simulink model "bh_explore_1dof_on_the_ROAD"  (R2026b)
settings: Solver=ode15s  StopTime=12  MaxStep=0.001  RelTol=1e-5  EnableMultiTasking=on
values from neighbouring files (symbols this model uses):
  s = saveObjectImpl@matlab.System(obj)    [bh_road_hump_A_SYSO.m]
undefined symbols (not defined in the file or in its folder): plant_T, X, Y, Z
libraries: sm_lib x5, nesl_utility x1
settings Model: Creator=smiller  LastModifiedBy=bhorton
settings DataIOCC: LimitDataPoints=on  ReturnWorkspaceOutputs=off  SaveFormat=Array
settings OptimizationCC: LifeSpan=inf
settings DebuggingCC: AllowSymbolicDim=off  ArithmeticOperatorsInVariantConditions=warning  MergeDetectMultiDrivingBlocksExec=none  SFExecutionAtInitializationDiag=none  SFNoUnconditionalDefaultTransitionDiag=warning  SFUnexpectedBacktrackingDiag=warning  SolverPrmCheckMsg=warning  StateNameClashWarn=warning  UnderspecifiedInitializationDetection=Classic
settings HardwareCC: ProdEndianess=Unspecified  ProdHWDeviceType=32-bit Generic  ProdIntDivRoundTo=Undefined  ProdLargestAtomicFloat=None
settings ModelReferenceCC: PropagateSignalLabelsOutOfModel=off
settings SFSimCC: CustomCodeUndefinedFunction=UseInterfaceOnly  SimUseLocalCustomCode=off
settings RTWCC: DLArmComputeVersion=19.05  RTWUseLocalCustomCode=off
settings CodeAppCC: StateflowObjectComments=on
settings GRTTargetCC: TargetLangStandard=C89/C90 (ANSI)
settings ConfigComp: CovExternalEMLEnable=off  CovSFcnEnable=off  CovSaveCumulativeToWorkspaceVar=on  CovSaveSingleToWorkspaceVar=on
settings SimscapeCC: SimscapeNormalizeSystem=off  SimscapeUseEnergyAccounting=off
settings ExplorerConfigSet: InternalSimMechanicsExplorerSettings=|
  | <ExplorerConfiguration>
  | 
  |   <canonicalview>default</canonicalview>
  | 
  |   <TilePanel>
  |     <TileInfo>
  |       <Tiles Columns="1" Count="1" Height="395" Rows="1" Width="675">
  |         <Row Weight="1"/>
  |         <Column Weight="1"/>
  |         <Tile Height="1" Width="1" X="0" Y="0"/>
  |       </Tiles>
  |     </TileInfo>
  |     <SceneInfo>
  |       <SceneViewer>
  |         <IsThisViewStd>
  |           <IsStandardView>off</IsStandardView>
  |           <StandardViewName>Front</StandardViewName>
  |         </IsThisViewStd>
  |         <BGColor>
  |           <R>0.60000002384185791</R>
  |           <G>0.60000002384185791</G>
  |           <B>0.60000002384185791</B>
  |           <A>1</A>
  |         </BGColor>
  |         <Camera>
  |           <DoPerspective>on</DoPerspective>
  |           <Position>
  |             <X>0</X>
  |             <Y>-4.9406564584124654e-324</Y>
  |             <Z>3</Z>
  |           </Position>
  |           <Center>
  |             <X>0</X>
  |             <Y>-4.9406564584124654e-324</Y>
  |             <Z>0</Z>
  |           </Center>
  |           <Up>
  |             <X>0</X>
  |             <Y>1</Y>
  |             <Z>0</Z>
  |           </Up>
  |           <XLim>1.3989229744649958</XLim>
  |           <YLim>1.3989229744649958</YLim>
  |           <ViewLimDist>0.01</ViewLimDist>
  |         </Camera>
  |       </SceneViewer>
  |     </SceneInfo>
  |   </TilePanel>
  | 
  |   <MechEditorPanel>
  |     <GfxPanelCameraMap>
  |       <MapElement CameraMLId="Camera1" GfxPanelIndex="0"/>
  |     </GfxPanelCameraMap>
  |     <Cameras>
  |       <Camera>
  |         <Id>Camera1</Id>
  |         <Value>
  |           <Name>Camera1</Name>
  |           <NativeCamera>
  |             <PositionTrackingFeature>CAR_SIMSCAPE.RF_CAM.R</PositionTrackingFeature>
  |             <CenterTrackingFeature>CAR_SIMSCAPE.Road.R</CenterTrackingFeature>
  |             <UpVectorTrackingFeature>CAR_SIMSCAPE.RF1.R</UpVectorTrackingFeature>
  |             <CenterTrackingOrigin>on</CenterTrackingOrigin>
  |             <UpVectorTrackingDirection>+Y</UpVectorTrackingDirection>
  |           </NativeCamera>
  |         </Value>
  |       </Camera>
  |     </Cameras>
  |     <VideoCreator>
  |       <IncludeTiles>All</IncludeTiles>
  |       <IncludeTime>off</IncludeTime>
  |       <IncludeWorldFrame>off</IncludeWorldFrame>
  |       <PlaybackSpeedRatio>2</PlaybackSpeedRatio>
  |       <FrameRate>30</FrameRate>
  |       <FrameSize>[400, 400]</FrameSize>
  |       <VideoFormat>MPEG4</VideoFormat>
  |     </VideoCreator>
  |   </MechEditorPanel>
  | 
  |   <PlaybackSettings>
  |     <PlaybackSpeedFactor>0.5</PlaybackSpeedFactor>
  |   </PlaybackSettings>
  | 
  | </ExplorerConfiguration>

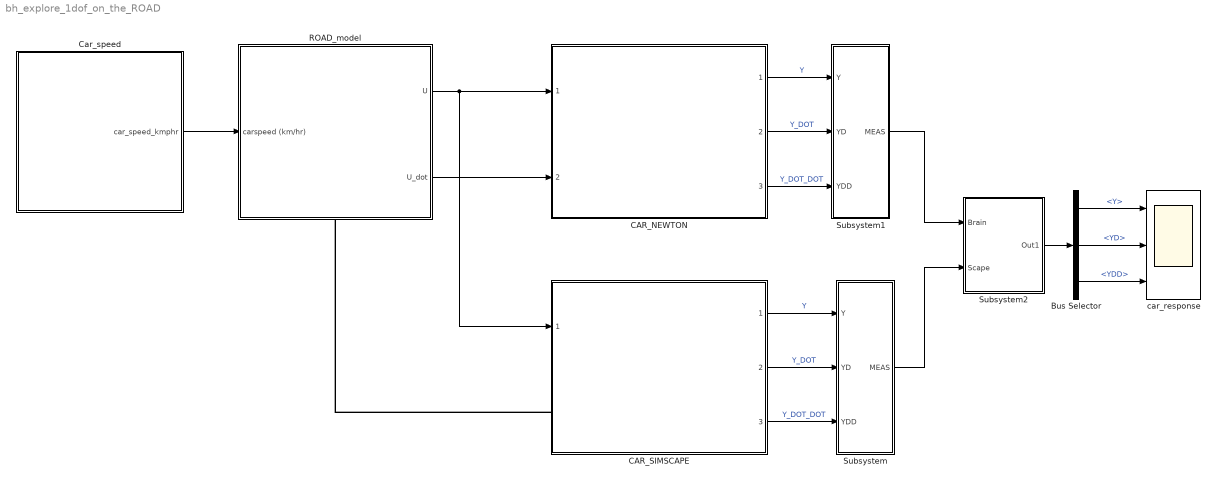
== system bh_explore_1dof_on_the_ROAD ==
  Bus Selector : BusSelector  OutputSignals=Y,YD,YDD
  CAR_NEWTON : Subsystem  ReferencedSubsystem=bh_COMPONENT_1dof_NEWTON  m=plant_T.m  c=plant_T.c  k=plant_T.k  y0=IC_T.y  y_dot_0=IC_T.y_dot
  CAR_SIMSCAPE : Subsystem  ReferencedSubsystem=bh_COMPONENT_1dof_SIMSCAPE  m=plant_T.m  c=plant_T.c  k=plant_T.k  L_EQ=IC_T.L_EQ  U_m_rel_R=IC_T.U_m_rel_R  U_m_rel_R_dot=IC_T.U_m_rel_R_dot
  Car_speed : Subsystem
  ROAD_model : Subsystem
      settings: PortSchema="{\"entries\":[{\"content\":{\"sides\":[{\"content\":{\"connectorIds\":[\"In1\"]},\"type\":\"ConnectorPlacement.EquallySpacedRectSide\",\"uuid\":\"1fb0e359-1d6f-495f-b416-4042b3ceba31\"},{\"content\":{\"connectorIds\":[\"Out1\",\"Out2\"],\"side\":\"RIGHT\"},\"type\":\"ConnectorPlacement.EquallySpacedRectSide\",\"uuid\":\"86004b89-795c-49b7-9809-342f6a5939d0\"},{\"content\":{\"side\":\"TOP\"},\"type\":\"ConnectorPlacement.EquallySpacedRectSide\",\"uuid\":\"63e39511-0cd1-4623-81a4-4c1485d2dba0\"},{\"content\":{\"connectorIds\":[\"RConn1\"],\"side\":\"BOTTOM\"},\"type\":\"ConnectorPlacement.EquallySpacedRectSide\",\"uuid\":\"6d6a2f3b-9911-4ef3-b1fe-c7ef6b98e3da\"}]},\"type\":\"ConnectorPlacement.EquallySpacedConnector\",\"uuid\":\"0b009940-cb7a-402d-bea6-65ae1d55ed5c\"}],\"packageUris\":[\"http://schema.mathworks.com/mf0/Connector/R2020b\"],\"version\":\"1.0\"}"
  Subsystem : Subsystem
  Subsystem1 : Subsystem
  Subsystem2 : Subsystem
  car_response : Scope  NumInputPorts=3
      settings: ActiveDisplayYMinimum=-0.2278214499400405  ActiveDisplayYMaximum=-0.13085171197243853  DataLoggingVariableName=ScopeData2
  wires:
  Car_speed/1(car_speed_kmphr) -> ROAD_model/1(carspeed (km/hr))
  Bus Selector/2 -> car_response/2  "<YD>"
  CAR_SIMSCAPE/2 -> Subsystem/2(YD)  "Y_DOT"
  CAR_NEWTON/1 -> Subsystem1/1(Y)  "Y"
  Subsystem2/1(Out1) -> Bus Selector/1
  Bus Selector/1 -> car_response/1  "<Y>"
  CAR_NEWTON/2 -> Subsystem1/2(YD)  "Y_DOT"
  CAR_SIMSCAPE/3 -> Subsystem/3(YDD)  "Y_DOT_DOT"
  CAR_NEWTON/3 -> Subsystem1/3(YDD)  "Y_DOT_DOT"
  CAR_SIMSCAPE/1 -> Subsystem/1(Y)  "Y"
  Bus Selector/3 -> car_response/3  "<YDD>"
  Subsystem1/1(MEAS) -> Subsystem2/1(Brain)
  Subsystem/1(MEAS) -> Subsystem2/2(Scape)
  ROAD_model/1(U) -> CAR_NEWTON/1, CAR_SIMSCAPE/1
  ROAD_model/2(U_dot) -> CAR_NEWTON/2
  connections:
  CAR_SIMSCAPE/LConn1 -- ROAD_model/RConn1

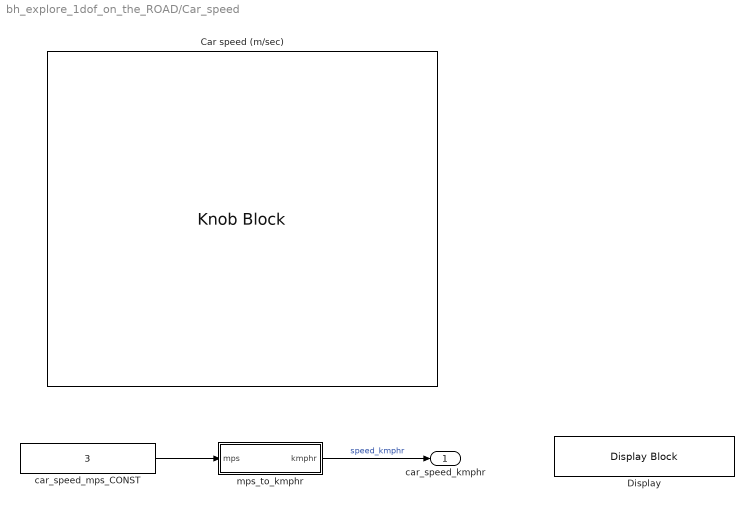
== system bh_explore_1dof_on_the_ROAD/Car_speed ==
  Car speed (m/sec) : KnobBlock  LabelPosition=Hide  ScaleMax=30  TickInterval=1
  Display : DisplayBlock  Transparency=1  GridColor=[0.502, 0.502, 0.502]
  car_speed_mps_CONST : Constant  Value=3
  mps_to_kmphr : Subsystem
  car_speed_kmphr : Outport
  wires:
  car_speed_mps_CONST/1 -> mps_to_kmphr/1(mps)
  mps_to_kmphr/1(kmphr) -> car_speed_kmphr/1  "speed_kmphr"

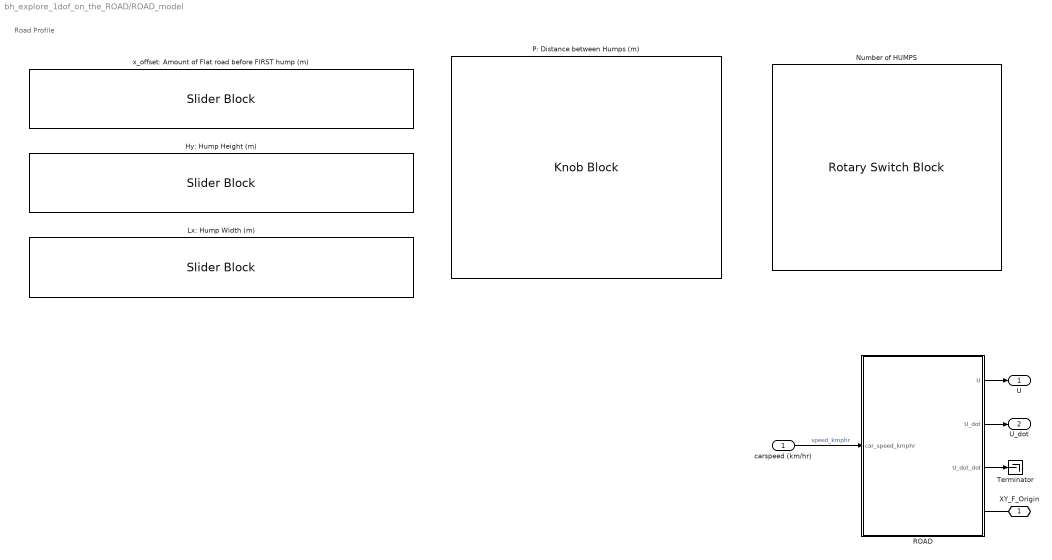
== system bh_explore_1dof_on_the_ROAD/ROAD_model ==
  note: Road Profile
  carspeed (km/hr) : Inport
  Hy: Hump Height (m) : SliderBlock  LabelPosition=Hide  ScaleMax=0.25
  Lx: Hump Width (m) : SliderBlock  LabelPosition=Hide  ScaleMax=1
  Number of HUMPS : RotarySwitchBlock  LabelPosition=Hide
  P: Distance between Humps (m) : KnobBlock  LabelPosition=Hide
  ROAD : Subsystem  mask{m_Hy=0.1981572234156821, m_Lx=1, m_P=9.707276629144626, m_x_offset=2, m_Np=20}
      mask prompts: m_Hy "Height of hump (m)"; m_Lx "Length of hump (m)"; m_P "Period of window (m)"; m_x_offset "X direction offset"; m_Np "Number of periods"
      mask init:
      | % create SYS object
      | OBJ = bh_road_hump_A_SYSO("Hy",m_Hy, "Lx",m_Lx, "P",m_P, ...
      |                           "x_offset",m_x_offset, "NUM_PERIODS",m_Np);
      |                       
      | tmp_x = linspace(0,(m_Np*m_P  +  m_x_offset), 1e4);
      | tmp_y = OBJ.get_y(tmp_x);
      | tmp_z = -2 * ones(size(tmp_x));
      | 
      | the_road_XYZ = [ tmp_x(:), tmp_y(:), tmp_z(:) ];
      mask DialogControl Control2 Prompt: Road Profile Parameters
  Terminator : Terminator
  x_offset: Amount of Flat road before FIRST hump (m) : SliderBlock  LabelPosition=Hide  ScaleMax=10
  XY_F_Origin : PMIOPort  Side=Right
  U : Outport
  U_dot : Outport  Port=2
  wires:
  ROAD/1(U) -> U/1
  ROAD/3(U_dot_dot) -> Terminator/1
  ROAD/2(U_dot) -> U_dot/1
  carspeed (km/hr)/1 -> ROAD/1(car_speed_kmphr)  "speed_kmphr"
  connections:
  XY_F_Origin/RConn1 -- ROAD/RConn1

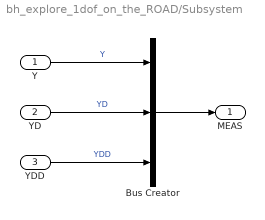
== system bh_explore_1dof_on_the_ROAD/Subsystem ==
  Y : Inport
  YD : Inport  Port=2
  YDD : Inport  Port=3
  Bus Creator : BusCreator  Inputs=3
  MEAS : Outport
  wires:
  YD/1 -> Bus Creator/2  "YD"
  YDD/1 -> Bus Creator/3  "YDD"
  Y/1 -> Bus Creator/1  "Y"
  Bus Creator/1 -> MEAS/1

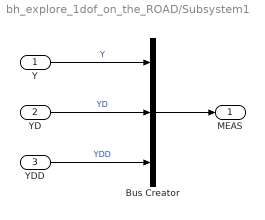
== system bh_explore_1dof_on_the_ROAD/Subsystem1 ==
  Y : Inport
  YD : Inport  Port=2
  YDD : Inport  Port=3
  Bus Creator : BusCreator  Inputs=3
  MEAS : Outport
  wires:
  YD/1 -> Bus Creator/2  "YD"
  YDD/1 -> Bus Creator/3  "YDD"
  Y/1 -> Bus Creator/1  "Y"
  Bus Creator/1 -> MEAS/1

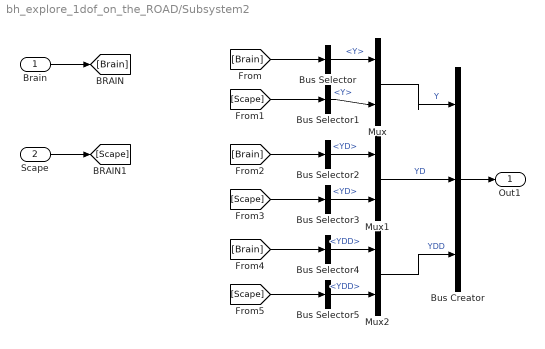
== system bh_explore_1dof_on_the_ROAD/Subsystem2 ==
  Brain : Inport
  Scape : Inport  Port=2
  Bus Creator : BusCreator  Inputs=3
  Bus Selector : BusSelector  OutputSignals=Y
  Bus Selector1 : BusSelector  OutputSignals=Y
  Bus Selector2 : BusSelector  OutputSignals=YD
  Bus Selector3 : BusSelector  OutputSignals=YD
  Bus Selector4 : BusSelector  OutputSignals=YDD
  Bus Selector5 : BusSelector  OutputSignals=YDD
  Mux : Mux  Inputs=2
  Mux1 : Mux  Inputs=2
  Mux2 : Mux  Inputs=2
  Out1 : Outport
  wires:
  Scape/1 -> [Scape]
  Brain/1 -> [Brain]
  [Brain] -> Bus Selector/1
  [Scape] -> Bus Selector1/1
  Bus Selector/1 -> Mux/1  "<Y>"
  Bus Selector1/1 -> Mux/2  "<Y>"
  Bus Selector2/1 -> Mux1/1  "<YD>"
  [Brain] -> Bus Selector2/1
  [Scape] -> Bus Selector3/1
  Bus Selector3/1 -> Mux1/2  "<YD>"
  Bus Selector4/1 -> Mux2/1  "<YDD>"
  [Brain] -> Bus Selector4/1
  [Scape] -> Bus Selector5/1
  Bus Selector5/1 -> Mux2/2  "<YDD>"
  Mux1/1 -> Bus Creator/2  "YD"
  Mux/1 -> Bus Creator/1  "Y"
  Mux2/1 -> Bus Creator/3  "YDD"
  Bus Creator/1 -> Out1/1

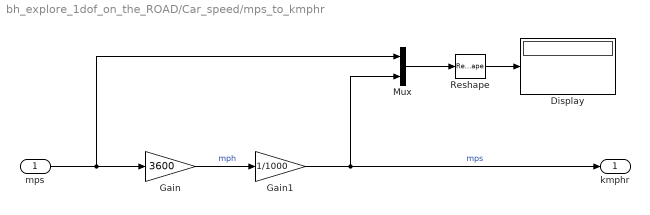
== system bh_explore_1dof_on_the_ROAD/Car_speed/mps_to_kmphr ==
  mps : Inport
  Display : Display
  Gain : Gain  Gain=3600
  Gain1 : Gain  Gain=1/1000
  Mux : Mux  Inputs=2
  Reshape : Reshape  OutputDimensionality=Column vector (2-D)
  kmphr : Outport
  wires:
  mps/1 -> Mux/1, Gain/1
  Gain/1 -> Gain1/1  "mph"
  Gain1/1 -> Mux/2, kmphr/1  "mps"
  Reshape/1 -> Display/1
  Mux/1 -> Reshape/1

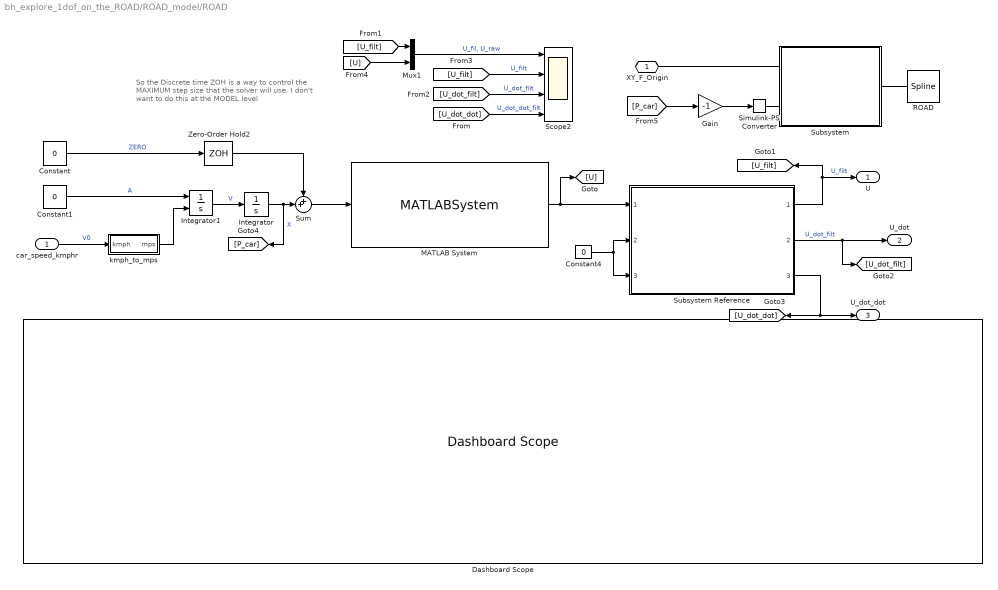
== system bh_explore_1dof_on_the_ROAD/ROAD_model/ROAD ==
  note: So the Discrete time ZOH is a way to control
      | the MAXIMUM step size that the solver will use.
      |
      | I don't want to do this at the MODEL level
  car_speed_kmphr : Inport
  Constant : Constant  Value=0
  Constant1 : Constant  Value=0
  Constant4 : Constant  Value=0
  Dashboard Scope : DashboardScope  FontColor=[0.0, 0.0, 0.0]
  Gain : Gain  Gain=-1
  Integrator : Integrator
  Integrator1 : Integrator  InitialConditionSource=external
  MATLAB System : MATLABSystem  System=bh_road_hump_A_SYSO  Hy=m_Hy  Lx=m_Lx  P=m_P  x_offset=m_x_offset  NUM_PERIODS=m_Np  SimulateUsing=Interpreted execution
      mask Type: bh_road_hump_A_SYSO
  Mux1 : Mux  Inputs=2
  ROAD : sm_lib/Curves and Surfaces/Spline  DataPoints=the_road_XYZ  DataPointsUnits=m  EndConditionType=Natural  GraphicType=FromGeometry  MarkerShape=Sphere  MarkerSize=10  GraphicVisPropType=SimpleVisualProperties  GraphicDiffuseColor=[0.2 1.0 0.2]  GraphicOpacity=1.0  GraphicSpecularColor=[0.5 0.5 0.5 1.0]  GraphicAmbientColor=[0.15 0.15 0.15 1.0]  GraphicEmissiveColor=[0.0 0.0 0.0 1.0]  GraphicShininess=75
  Scope2 : Scope  NumInputPorts=4
      settings: ActiveDisplayYMinimum=-0.01  ActiveDisplayYMaximum=0.09
  Simulink-PS Converter : nesl_utility/Simulink-PS Converter  PhysicalDomain=network_engine_domain  SubClassName=ps_input  LeftPortType=input  RightPortType=output  PseudoPeriodic=off  Frequencies=[]  NoiseDistribution=none  NoiseParameters=[]  Unit=m  AffineConversion=off  FilteringAndDerivatives=filter  SimscapeFilterOrder=2  InputFilterTimeConstant=0.001  UdotUserProvided=0
  Subsystem : Subsystem
  Subsystem Reference : Subsystem  ReferencedSubsystem=bh_COMPONENT_deriv_est  wn=2*pi*1000  p=1
  Sum : Sum  Inputs=++|
  Zero-Order Hold2 : ZeroOrderHold  SampleTime=1/1000
      settings: AttributesFormatString=dT =%<SampleTime>
  kmph_to_mps : Subsystem
  XY_F_Origin : PMIOPort  Side=Right
  U : Outport
  U_dot : Outport  Port=2
  U_dot_dot : Outport  Port=3
  wires:
  Integrator/1 -> [P_car], Sum/2  "X"
  Mux1/1 -> Scope2/1  "U_fil, U_raw"
  Sum/1 -> MATLAB System/1
  Constant1/1 -> Integrator1/1  "A"
  Constant/1 -> Zero-Order Hold2/1  "ZERO"
  MATLAB System/1 -> [U], Subsystem Reference/1
  Integrator1/1 -> Integrator/1  "V"
  kmph_to_mps/1(mps) -> Integrator1/2
  car_speed_kmphr/1 -> kmph_to_mps/1(kmph)  "V0"
  Zero-Order Hold2/1 -> Sum/1
  Constant4/1 -> Subsystem Reference/3, Subsystem Reference/2
  Subsystem Reference/2 -> U_dot/1, [U_dot_filt]  "U_dot_filt"
  Subsystem Reference/1 -> U/1, [U_filt]  "U_filt"
  [U] -> Mux1/2
  [U_filt] -> Mux1/1
  [U_filt] -> Scope2/2  "U_filt"
  [U_dot_filt] -> Scope2/3  "U_dot_filt"
  Subsystem Reference/3 -> U_dot_dot/1, [U_dot_dot]
  [U_dot_dot] -> Scope2/4  "U_dot_dot_filt"
  [P_car] -> Gain/1
  Gain/1 -> Simulink-PS Converter/1
  connections:
  Subsystem/LConn1 -- XY_F_Origin/RConn1
  Simulink-PS Converter/RConn1 -- Subsystem/LConn2
  ROAD/LConn1 -- Subsystem/RConn1

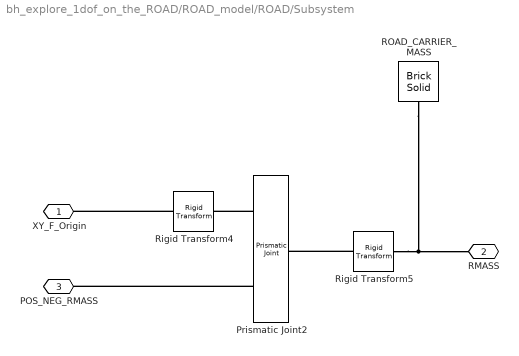
== system bh_explore_1dof_on_the_ROAD/ROAD_model/ROAD/Subsystem ==
  Prismatic Joint2 : sm_lib/Joints/Prismatic Joint  JointMode=Normal  CompositeWrenchDir=FollowerOnBase  CompositeWrenchFrame=BaseFrame  SenseConstraintForce=off  SenseConstraintTorque=off  SenseTotalForce=off  SenseTotalTorque=off  PositionTargetSpecify=off  PositionTargetPriority=High  PositionTargetValue=0  PositionTargetValueUnits=m  VelocityTargetSpecify=off  VelocityTargetPriority=High  VelocityTargetValue=0  VelocityTargetValueUnits=m/s  EquilibriumPosition=0  EquilibriumPositionUnits=m  SpringStiffness=0  SpringStiffnessUnits=N/m  DampingCoefficient=0  DampingCoefficientUnits=N/(m/s)  LowerLimitSpecify=off  LowerLimitBound=-1  LowerLimitBoundUnits=m  LowerLimitStiffness=1e6  LowerLimitStiffnessUnits=N/m  LowerLimitDamping=1e3  LowerLimitDampingUnits=N/(m/s)  LowerLimitTransitionRegionWidth=1e-4  LowerLimitTransitionRegionWidthUnits=m  UpperLimitSpecify=off  UpperLimitBound=1  UpperLimitBoundUnits=m  UpperLimitStiffness=1e6  UpperLimitStiffnessUnits=N/m  UpperLimitDamping=1e3  UpperLimitDampingUnits=N/(m/s)  UpperLimitTransitionRegionWidth=1e-4  UpperLimitTransitionRegionWidthUnits=m  TorqueActuationMode=ComputedTorque  MotionActuationMode=InputMotion  SensePosition=off  SenseVelocity=off  SenseAcceleration=off  SenseTorqueForce=off  SenseLowerLimitTorqueForce=off  SenseUpperLimitTorqueForce=off
  ROAD_CARRIER_MASS : sm_lib/Body Elements/Brick Solid  BrickDimensions=[1, 1, 1]/100  BrickDimensionsUnits=m  ExportEntireGeometry=off  InertiaType=PointMass  BasedOnType=Density  Density=1000  DensityUnits=kg/m^3  Mass=1  MassUnits=kg  CenterOfMass=[0 0 0]  CenterOfMassUnits=m  MomentsOfInertia=[1 1 1]  MomentsOfInertiaUnits=kg*m^2  ProductsOfInertia=[0 0 0]  ProductsOfInertiaUnits=kg*m^2  GraphicType=FromGeometry  MarkerShape=Sphere  MarkerSize=10  GraphicVisPropType=SimpleVisualProperties  GraphicDiffuseColor=[0.0 0.8 0.2]  GraphicOpacity=1.0  GraphicSpecularColor=[0.5 0.5 0.5 1.0]  GraphicAmbientColor=[0.15 0.15 0.15 1.0]  GraphicEmissiveColor=[0.0 0.0 0.0 1.0]  GraphicShininess=75  DoExposeReferenceFrame=on  SerializedFrames=<Frames/>
  Rigid Transform4 : sm_lib/Frames and Transforms/Rigid Transform  RotationMethod=AlignedAxes  FollAlignAxisA=+Z  BaseAlignAxisA=+X  FollAlignAxisB=+Y  BaseAlignAxisB=+Y  RotationStandardAxis=+Z  RotationAngle=0.0  RotationAngleUnits=deg  RotationArbitraryAxis=[0 0 1]  RotationSequenceAxes=FollowerAxes  RotationSequence=XYX  RotationSequenceAngles=[0 0 0]  RotationSequenceAnglesUnits=deg  RotationMatrix=[1 0 0; 0 1 0; 0 0 1]  Quaternion=[1 0 0 0]  TranslationMethod=None  TranslationCartesianOffset=[0 0 0]  TranslationCartesianOffsetUnits=m  TranslationStandardAxis=+Z  TranslationStandardOffset=0  TranslationStandardOffsetUnits=m  TranslationROffset=0  TranslationROffsetUnits=m  TranslationThetaOffset=0  TranslationThetaOffsetUnits=deg  TranslationZOffset=0  TranslationZOffsetUnits=m
  Rigid Transform5 : sm_lib/Frames and Transforms/Rigid Transform  RotationMethod=AlignedAxes  FollAlignAxisA=+X  BaseAlignAxisA=+Z  FollAlignAxisB=+Y  BaseAlignAxisB=+Y  RotationStandardAxis=+Z  RotationAngle=0.0  RotationAngleUnits=deg  RotationArbitraryAxis=[0 0 1]  RotationSequenceAxes=FollowerAxes  RotationSequence=XYX  RotationSequenceAngles=[0 0 0]  RotationSequenceAnglesUnits=deg  RotationMatrix=[1 0 0; 0 1 0; 0 0 1]  Quaternion=[1 0 0 0]  TranslationMethod=None  TranslationCartesianOffset=[0 0 0]  TranslationCartesianOffsetUnits=m  TranslationStandardAxis=+Z  TranslationStandardOffset=0  TranslationStandardOffsetUnits=m  TranslationROffset=0  TranslationROffsetUnits=m  TranslationThetaOffset=0  TranslationThetaOffsetUnits=deg  TranslationZOffset=0  TranslationZOffsetUnits=m
  XY_F_Origin : PMIOPort  Side=Left
  RMASS : PMIOPort  Port=2  Side=Right
  POS_NEG_RMASS : PMIOPort  Port=3  Side=Left
  connections:
  Prismatic Joint2/LConn1 -- Rigid Transform4/RConn1
  Rigid Transform5/LConn1 -- Prismatic Joint2/RConn1
  Prismatic Joint2/LConn2 -- POS_NEG_RMASS/RConn1
  Rigid Transform4/LConn1 -- XY_F_Origin/RConn1
  Rigid Transform5/RConn1 -- ROAD_CARRIER_MASS/RConn1 -- RMASS/RConn1

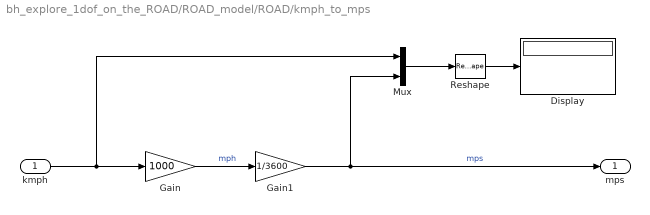
== system bh_explore_1dof_on_the_ROAD/ROAD_model/ROAD/kmph_to_mps ==
  kmph : Inport
  Display : Display
  Gain : Gain  Gain=1000
  Gain1 : Gain  Gain=1/3600
  Mux : Mux  Inputs=2
  Reshape : Reshape  OutputDimensionality=Column vector (2-D)
  mps : Outport
  wires:
  kmph/1 -> Mux/1, Gain/1
  Gain/1 -> Gain1/1  "mph"
  Gain1/1 -> Mux/2, mps/1  "mps"
  Reshape/1 -> Display/1
  Mux/1 -> Reshape/1
